simulink model "controller_tuning"  (R2024b)
settings: Solver=FixedStepAuto  StartTime=0.0  StopTime=inf  FixedStep=0.001  RelTol=1e-3
undefined symbols (not defined in the file): drawaircraft, drawaircraft2, force_moment, MAV, position_rhombus, sample_time, SIM
libraries: slpidlib x12
(part 2 of 2)

== system controller_tuning/plant/6DOF dynamics ==
  f,m : Inport
  S-Function : S-Function  FunctionName=UAVdynamics  Parameters=MAV  SFunctionDeploymentMode=off  EnableBusSupport=off
  state : Outport
  F,M : Outport  Port=2
  wires:
  S-Function/1 -> state/1  "state"
  f,m/1 -> S-Function/1, F,M/1

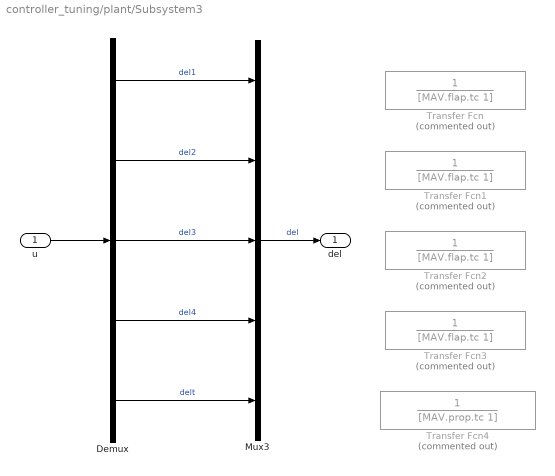
== system controller_tuning/plant/Subsystem3 ==
  u : Inport
  Demux : Demux  Outputs=5
  Mux3 : Mux  Inputs=5
  Transfer Fcn{,1..3} (4 alike) : TransferFcn  Commented=on  Denominator=[MAV.flap.tc 1]
  Transfer Fcn4 : TransferFcn  Commented=on  Denominator=[MAV.prop.tc 1]
  del : Outport
  wires:
  Mux3/1 -> del/1  "del"
  Demux/1 -> Mux3/1  "del1"
  Demux/2 -> Mux3/2  "del2"
  Demux/4 -> Mux3/4  "del4"
  Demux/3 -> Mux3/3  "del3"
  Demux/5 -> Mux3/5  "delt"
  u/1 -> Demux/1

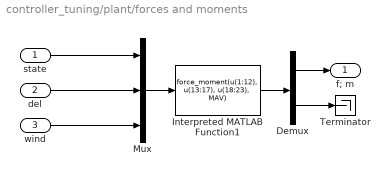
== system controller_tuning/plant/forces and moments ==
  state : Inport
  del : Inport  Port=2
  wind : Inport  Port=3
  Demux : Demux  Outputs=[6,3]
  Interpreted MATLAB Function1 : MATLABFcn  MATLABFcn=force_moment(u(1:12), u(13:17), u(18:23), MAV)  OutputDimensions=9
  Mux : Mux  Inputs=3
  Terminator : Terminator
  f; m : Outport
  wires:
  Demux/2 -> Terminator/1
  Demux/1 -> f; m/1
  Interpreted MATLAB Function1/1 -> Demux/1
  wind/1 -> Mux/3
  del/1 -> Mux/2
  state/1 -> Mux/1
  Mux/1 -> Interpreted MATLAB Function1/1

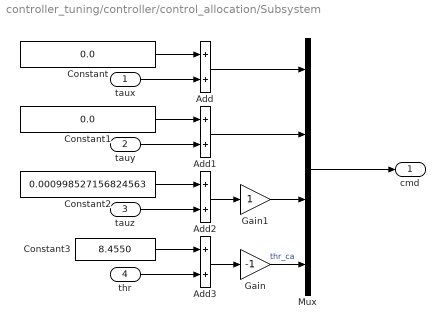
== system controller_tuning/controller/control_allocation/Subsystem ==
  taux : Inport
  tauy : Inport  Port=2
  tauz : Inport  Port=3
  thr : Inport  Port=4
  Add{,1..3} (4 alike) : Sum
  Constant : Constant  Value=0.0
  Constant1 : Constant  Value=0.0
  Constant2 : Constant  Value=0.000998527156824563
  Constant3 : Constant  Value=8.4550
  Gain : Gain  Gain=-1
  Gain1 : Gain
  Mux : Mux
  cmd : Outport
  wires:
  taux/1 -> Add/2
  Add2/1 -> Gain1/1
  Constant/1 -> Add/1
  Mux/1 -> cmd/1
  Add1/1 -> Mux/2
  Add/1 -> Mux/1
  Constant1/1 -> Add1/1
  tauy/1 -> Add1/2
  tauz/1 -> Add2/2
  Constant2/1 -> Add2/1
  Add3/1 -> Gain/1
  thr/1 -> Add3/2
  Constant3/1 -> Add3/1
  Gain/1 -> Mux/4  "thr_ca"
  Gain1/1 -> Mux/3

== matlab function controller_tuning/controller/position//velocity controller/MATLAB Function1 ==
  data: psi input; R output
function R = R_psi(psi)
    R = [cos(psi), sin(psi);
        -sin(psi), cos(psi)];
end

== matlab function controller_tuning/controller/control_allocation/MATLAB Function ==
  data: fm input; deltas output; MAV input; prev_delt input
function deltas   = control_allocation(fm, MAV, prev_delt)
    % desired_forces_moments = [Mx; My; Mz; Fz]
    
    volt_prev = MAV.prop_data.volt_max * prev_delt;
    [T1, tau1] = prop_second_order(0, volt_prev, MAV);
    v_flap = sqrt(T1 / (2 * MAV.rho * MAV.prop_data.prop_area));
    
    q = 0.5 * MAV.rho * (v_flap^2); 
    C_lift = q * MAV.flap.s * MAV.flap.cla;
    
    K_T = T1 / prev_delt;
    K_Q = tau1 / prev_delt;

    % Mapping: [d1, d2, d3, d4, dt] -> [Mx, My, Mz, Fz]
    xt = MAV.flap.xt; yt = MAV.flap.yt; zt = MAV.flap.zt;
    
    B = [ ...
        (-zt*C_lift),  0,            (-zt*C_lift), 0,            0;
        0,             (-zt*C_lift), 0,            (-zt*C_lift), 0;
        (xt*C_lift),   (-yt*C_lift), (-xt*C_lift), (yt*C_lift),  K_Q;
        0,             0,            0,            0,            -K_T;
    ];
    
    % Pseudo Inverse
    P = pinv(B);
    
    % Raw Actuator Commands
    deltas = P * fm;
end

== matlab function controller_tuning/controller/position//velocity controller/MATLAB Function ==
  data: phi input; R output; theta input; psi input
function R = rotate_inter2body(phi, theta, psi)
    R_psi = [cos(psi), sin(psi), 0;
            -sin(psi), cos(psi), 0
            0, 0, 1];
    R_theta = [cos(theta), 0, -sin(theta);
                0 , 1, 0;
                sin(theta), 0, cos(theta)];
    R_phi = [1, 0, 0;
             0, cos(phi), sin(phi);
             0, -sin(phi), cos(phi)];
    R = R_phi * R_theta * R_psi;
end
